simulink model "sim_active_hc_hlsii"  (R2020b)
settings: Solver=VariableStepAuto  StartTime=0.0  StopTime=10.0  RelTol=1e-3
InitFcn:
  | %————————————————————————————
  | %自变量
  | %————————————————————————————
  | IB = 300/1000;
  | fF = -90/180*pi;
  | X = 0;
  | thetaL = -0/180*pi;
  | thetaLH = -0/180*pi;
  | wa = 2*pi*1e3;
  | wp = 2*pi*1e3;
  | waH = 2*pi*2e3;
  | wpH = 2*pi*1e3;
  | KCa = 30;
  | KCp = 50;
  | KCaH = 10;
  | KCpH = 30;
  | %————————————————————————————
  | %常量（不同模式不同）
  | %————————————————————————————
  | VC = 250e3;
  | %————————————————————————————
  | %常量
  | %————————————————————————————
  | beta = 2;
  | betaH = 2;
  | RL0 = 2*3.3e6;
  | RLH0 = 2*2.5e6;
  | Q0 = 28000;
  | QH0 = 18000;
  | RL = RL0/(1+beta);
  | RLH = RLH0/(1+betaH);
  | QL = Q0/(1+beta);
  | QLH = QH0/(1+betaH);
  | n = 4;
  | frf = 204e6;
  | fhrf = frf*n;
  | U_ratio_e =16.73e3;
  | RL_ratio_QL = QL/RL;
  | RLH_ratio_QLH = QLH/RLH;
  | sigma = 2*pi*frf/(2*QL);
  | sigmaH = 2*pi*fhrf/(2*QLH);
  | DRFB_delay = 1e-6;
  | mc_loop_delay = 1e-6;
  | hc_loop_delay = 1e-6;
  | %————————————————————————————
  | %计算得出以下物理量
  | %————————————————————————————
  | k = sqrt(1/n/n-(U_ratio_e/VC)^2/(n^2-1));
  | VH = k*VC;
  | Gf = X/RL;
  | I0 = VC/RL;
  | I0H = VH/RLH;
  | Y = IB/I0;
  | YH = IB/I0H;
  | fH = pi/2 - atan(n*U_ratio_e/VC/sqrt((n^2-1)^2-(U_ratio_e*n*n/VC)^2));
  | fs = pi/2 - asin(n*n*U_ratio_e/(n*n-1)/VC);
  | fLH = atan(tan(thetaLH)-YH*tan(thetaLH)*cos(fH)+YH*sin(fH));
  | %fL = atan(IB*tan(thetaL)*cos(fs)/I0+tan(thetaL)-IB*sin(fs)/I0);
  | %FL = atan(tan(fL)+X*(sin(fF)-cos(fF)*tan(fL)));
  | fL = -atan(Y*sin(fs)-X*sin(fF)-(1+Y*cos(fs)-X*cos(fF))*tan(thetaL));
  | thetaT = -atan((VC*cos(fs)-VH*cos(fH))/(VC*sin(fs)-VH*sin(fH)));
  | VT = sqrt(VC^2+VH^2-2*VC*VH*cos(fs-fH));
  | T0 = 1/(204e6/45);
  | ws = sqrt(2*pi*(4.7e-4)*45*VT*cos(-thetaT)/T0/T0/0.8/1e9);
  | alpha = U_ratio_e/T0/0.8/1e9;
  | %————————————————————————————
  | %传递函数各分子分母
  | %————————————————————————————
  | syms s
  | %sdelay = 1-s*DRFB_delay+s^2*DRFB_delay^2/2-s^3*DRFB_delay^3/6+s^4*DRFB_delay^4/24;
  | sdelay = 1-s*DRFB_delay;
  | G_fenmu = s^2+2*sigma*s+sigma^2*(sec(fL))^2;
  | Gaa_fenzi = sigma*s+sigma^2*(1+(tan(fL))^2);
  | Gpp_fenzi = Gaa_fenzi;
  | Gpa_fenzi = sigma*tan(fL)*s;
  | Gap_fenzi = -Gpa_fenzi;
  | Gaa = Gaa_fenzi/G_fenmu;
  | Gpp = Gpp_fenzi/G_fenmu;
  | Gpa = Gpa_fenzi/G_fenmu;
  | Gap = Gap_fenzi/G_fenmu;
  | IT = I0/cos(fL);
  | IG = I0*(1-X*cos(fF)+Y*cos(fs))/cos(thetaL);
  | GppB = IB/IT*(-Gap*sin(fs-fL)-Gpp*cos(fs-fL));
  | GpaB = IB/IT*(-Gaa*sin(fs-fL)-Gpa*cos(fs-fL));
  | GppG = IG/IT*(Gap*sin(thetaL-fL)+Gpp*cos(thetaL-fL));
  | GpaG = IG/IT*(Gaa*sin(thetaL-fL)+Gpa*cos(thetaL-fL));
  | GaaG = GppG;GapG = -GpaG;
  | GppF = X*IB/IT*(Gap*sin(fF-fL)+Gpp*cos(fF-fL));
  | GpaF = X*IB/IT*(Gaa*sin(fF-fL)+Gpa*cos(fF-fL));
  | GaaF = GppF;GapF = -GpaF;
  | [GppB_fenzi,GppB_fenmu] = numden(GppB);[GpaB_fenzi,GpaB_fenmu] = numden(GpaB);
  | [GppG_fenzi,GppG_fenmu] = numden(GppG);[GpaG_fenzi,GpaG_fenmu] = numden(GpaG);
  | [GaaG_fenzi,GaaG_fenmu] = numden(GaaG);[GapG_fenzi,GapG_fenmu] = numden(GapG);
  | [GppF_fenzi,GppF_fenmu] = numden(GppF);[GpaF_fenzi,GpaF_fenmu] = numden(GpaF);
  | [GaaF_fenzi,GaaF_fenmu] = numden(GaaF);[GapF_fenzi,GapF_fenmu] = numden(GapF);
  | GppB_fz = sym2poly(GppB_fenzi);GppB_fm = sym2poly(GppB_fenmu);
  | GpaB_fz = sym2poly(GpaB_fenzi);GpaB_fm = sym2poly(GpaB_fenmu);
  | GppG_fz = sym2poly(GppG_fenzi);GppG_fm = sym2poly(GppG_fenmu);
  | GpaG_fz = sym2poly(GpaG_fenzi);GpaG_fm = sym2poly(GpaG_fenmu);
  | GaaG_fz = sym2poly(GaaG_fenzi);GaaG_fm = sym2poly(GaaG_fenmu);
  | GapG_fz = sym2poly(GapG_fenzi);GapG_fm = sym2poly(GapG_fenmu);
  | GppF_fz = sym2poly(GppF_fenzi);GppF_fm = sym2poly(GppF_fenmu);
  | GpaF_fz = sym2poly(GpaF_fenzi);GpaF_fm = sym2poly(GpaF_fenmu);
  | GaaF_fz = sym2poly(GaaF_fenzi);GaaF_fm = sym2poly(GaaF_fenmu);
  | GapF_fz = sym2poly(GapF_fenzi);GapF_fm = sym2poly(GapF_fenmu);
  | 
  | GppH = (s*sigmaH+sigmaH^2*(1+(tan(fLH))^2))/(s^2+2*sigmaH*s+sigmaH^2*(1+(tan(fLH))^2));
  | GpaH = (s*sigmaH*tan(fLH))/(s^2+2*sigmaH*s+sigmaH^2*(1+(tan(fLH))^2));
  | GaaH = GppH;GapH = -GpaH;
  | ITH = I0H/cos(fLH);
  | IGH = I0H*(1-YH*cos(fH))/cos(thetaLH);
  | GppBH = IB/ITH*(GapH*sin(fH-fLH)+GppH*cos(fH-fLH));
  | GpaBH = IB/ITH*(GaaH*sin(fH-fLH)+GpaH*cos(fH-fLH));
  | GppGH = IGH/ITH*(GapH*sin(thetaLH-fLH)+GppH*cos(thetaLH-fLH));
  | GpaGH = IGH/ITH*(GaaH*sin(thetaLH-fLH)+GpaH*cos(thetaLH-fLH)) ;
  | GaaGH = GppGH;GapGH = -GpaGH;
  | [GppBH_fenzi,GppBH_fenmu] = numden(GppBH);[GpaBH_fenzi,GpaBH_fenmu] = numden(GpaBH);
  | [GppGH_fenzi,GppGH_fenmu] = numden(GppGH);[GpaGH_fenzi,GpaGH_fenmu] = numden(GpaGH);
  | [GaaGH_fenzi,GaaGH_fenmu] = numden(GaaGH);[GapGH_fenzi,GapGH_fenmu] = numden(GapGH);
  | GppBH_fz = sym2poly(GppBH_fenzi);GppBH_fm = sym2poly(GppBH_fenmu);
  | GpaBH_fz = sym2poly(GpaBH_fenzi);GpaBH_fm = sym2poly(GpaBH_fenmu);
  | GppGH_fz = sym2poly(GppGH_fenzi);GppGH_fm = sym2poly(GppGH_fenmu);
  | GpaGH_fz = sym2poly(GpaGH_fenzi);GpaGH_fm = sym2poly(GpaGH_fenmu);
  | GaaGH_fz = sym2poly(GaaGH_fenzi);GaaGH_fm = sym2poly(GaaGH_fenmu);
  | GapGH_fz = sym2poly(GapGH_fenzi);GapGH_fm = sym2poly(GapGH_fenmu);
  | 
  | B_fm = [1 alpha ws^2];
  | Cp_fz = wp;Cp_fm = [1 wp];
  | Ca_fz = wa;Ca_fm = [1 wa];
  | CpH_fz = wpH;CpH_fm = [1 wpH];
  | CaH_fz = waH;CaH_fm = [1 waH];
  | %————————————————————————————
  | %传递函数计算
  | %————————————————————————————
  | B = tf(ws^2,B_fm);
  | Cp = tf(Cp_fz,Cp_fm);Ca = tf(Ca_fz,Ca_fm);
  | GpaB = tf(GpaB_fz,GpaB_fm);GppB = tf(GppB_fz,GppB_fm);
  | GpaG = tf(GpaG_fz,GpaG_fm);GppG = tf(GppG_fz,GppG_fm);GapG = tf(GapG_fz,GapG_fm);GaaG = tf(GaaG_fz,GaaG_fm);
  | GpaF = tf(GpaF_fz,GpaF_fm);GppF = tf(GppF_fz,GppF_fm);GapF = tf(GapF_fz,GapF_fm);GaaF = tf(GaaF_fz,GaaF_fm);
  | GpaBH = tf(GpaBH_fz,GpaBH_fm);GppBH = tf(GppBH_fz,GppBH_fm);
  | GpaGH = tf(GpaGH_fz,GpaGH_fm);GppGH = tf(GppGH_fz,GppGH_fm);GapGH = tf(GapGH_fz,GapGH_fm);GaaGH = tf(GaaGH_fz,GaaGH_fm);
  | Gab = (-cos(thetaT-fs)-sin(thetaT-fs)*tan(thetaT))*VC/VT;
  | Gpb = (-sin(thetaT-fs)+cos(thetaT-fs)*tan(thetaT))*VC/VT;
  | GabH = (cos(thetaT-fH)+sin(thetaT-fH)*tan(thetaT))*VH/VT;
  | GpbH = (sin(thetaT-fH)-cos(thetaT-fH)*tan(thetaT))*VH/VT;
settings Model: Creator=Administrator  LastModifiedBy=Administrator
settings SFSimCC: CustomCodeUndefinedFunction=UseInterfaceOnly

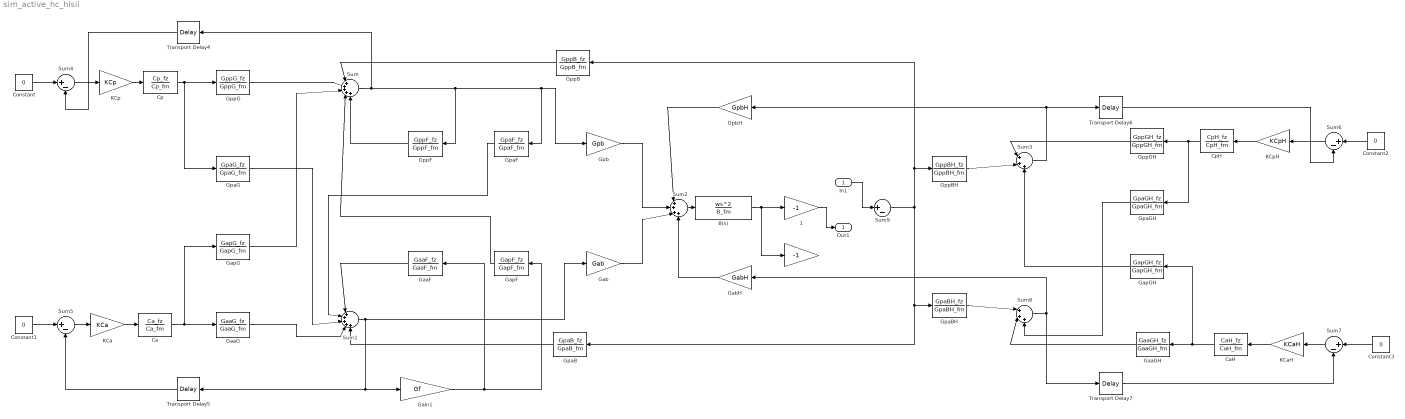
== system sim_active_hc_hlsii ==
  In1 : Inport
  "  " : Gain  Gain=-1
  "  1" : Gain  Gain=-1
  B(s) : TransferFcn  Numerator=ws^2  Denominator=B_fm
  Ca : TransferFcn  Numerator=Ca_fz  Denominator=Ca_fm
  CaH : TransferFcn  Numerator=CaH_fz  Denominator=CaH_fm
  Constant{,1..3} (4 alike) : Constant  Value=0
  Cp : TransferFcn  Numerator=Cp_fz  Denominator=Cp_fm
  CpH : TransferFcn  Numerator=CpH_fz  Denominator=CpH_fm
  GaaF : TransferFcn  Numerator=GaaF_fz  Denominator=GaaF_fm
  GaaG : TransferFcn  Numerator=GaaG_fz  Denominator=GaaG_fm
  GaaGH : TransferFcn  Numerator=GaaGH_fz  Denominator=GaaGH_fm
  Gab : Gain  Gain=Gab
  GabH : Gain  Gain=GabH
  Gain1 : Gain  Gain=Gf
  GapF : TransferFcn  Numerator=GapF_fz  Denominator=GapF_fm
  GapG : TransferFcn  Numerator=GapG_fz  Denominator=GapG_fm
  GapGH : TransferFcn  Numerator=GapGH_fz  Denominator=GapGH_fm
  GpaB : TransferFcn  Numerator=GpaB_fz  Denominator=GpaB_fm
  GpaBH : TransferFcn  Numerator=GpaBH_fz  Denominator=GpaBH_fm
  GpaF : TransferFcn  Numerator=GpaF_fz  Denominator=GpaF_fm
  GpaG : TransferFcn  Numerator=GpaG_fz  Denominator=GpaG_fm
  GpaGH : TransferFcn  Numerator=GpaGH_fz  Denominator=GpaGH_fm
  Gpb : Gain  Gain=Gpb
  GpbH : Gain  Gain=GpbH
  GppB : TransferFcn  Numerator=GppB_fz  Denominator=GppB_fm
  GppBH : TransferFcn  Numerator=GppBH_fz  Denominator=GppBH_fm
  GppF : TransferFcn  Numerator=GppF_fz  Denominator=GppF_fm
  GppG : TransferFcn  Numerator=GppG_fz  Denominator=GppG_fm
  GppGH : TransferFcn  Numerator=GppGH_fz  Denominator=GppGH_fm
  KCa : Gain  Gain=KCa
  KCaH : Gain  Gain=KCaH
  KCp : Gain  Gain=KCp
  KCpH : Gain  Gain=KCpH
  Sum : Sum  Inputs=|+++++
  Sum1 : Sum  Inputs=|+++++
  Sum2 : Sum  Inputs=|++++
  Sum3 : Sum  Inputs=|+++
  Sum{4..7,9} (5 alike) : Sum  Inputs=|+-
  Sum8 : Sum  Inputs=|+++
  Transport Delay4 : TransportDelay  DelayTime=mc_loop_delay
  Transport Delay5 : TransportDelay  DelayTime=mc_loop_delay
  Transport Delay6 : TransportDelay  DelayTime=hc_loop_delay
  Transport Delay7 : TransportDelay  DelayTime=hc_loop_delay
  Out1 : Outport
  wires:
  Ca/1 -> GaaG/1, GapG/1
  Sum4/1 -> KCp/1
  B(s)/1 -> "  1"/1, "  "/1
  GpaB/1 -> Sum1/5
  GaaG/1 -> Sum1/4
  Sum5/1 -> KCa/1
  GpbH/1 -> Sum2/1
  Cp/1 -> GpaG/1, GppG/1
  Gab/1 -> Sum2/3
  GppF/1 -> Sum/5
  GabH/1 -> Sum2/4
  Gpb/1 -> Sum2/2
  GapF/1 -> Sum/4
  GpaF/1 -> Sum1/2
  GapG/1 -> Sum/3
  GppG/1 -> Sum/2
  Gain1/1 -> GaaF/1, GapF/1
  GpaG/1 -> Sum1/3
  Sum/1 -> Transport Delay4/1, Gpb/1, GpaF/1, GppF/1
  Constant1/1 -> Sum5/1
  GaaF/1 -> Sum1/1
  Sum2/1 -> B(s)/1
  GppB/1 -> Sum/1
  Constant/1 -> Sum4/1
  Constant2/1 -> Sum6/1
  Constant3/1 -> Sum7/1
  Sum3/1 -> Transport Delay6/1, GpbH/1
  Sum8/1 -> Transport Delay7/1, GabH/1
  Sum7/1 -> KCaH/1
  CaH/1 -> GapGH/1, GaaGH/1
  GapGH/1 -> Sum3/3
  CpH/1 -> GpaGH/1, GppGH/1
  GpaGH/1 -> Sum8/3
  GaaGH/1 -> Sum8/2
  GppGH/1 -> Sum3/1
  GppBH/1 -> Sum3/2
  GpaBH/1 -> Sum8/1
  Sum1/1 -> Gab/1, Gain1/1, Transport Delay5/1
  KCa/1 -> Ca/1
  KCp/1 -> Cp/1
  Transport Delay4/1 -> Sum4/2
  Transport Delay5/1 -> Sum5/2
  Sum6/1 -> KCpH/1
  KCpH/1 -> CpH/1
  KCaH/1 -> CaH/1
  Transport Delay6/1 -> Sum6/2
  Transport Delay7/1 -> Sum7/2
  In1/1 -> Sum9/1
  Sum9/1 -> GpaB/1, GpaBH/1, GppB/1, GppBH/1
  "  1"/1 -> Out1/1
